simulink model "ackerman_ROS_controller_obstaculos_neuro_2022"  (R2022b)
settings: Solver=FixedStepDiscrete  StartTime=0.0  StopTime=120  FixedStep=0.1  RelTol=1e-3
undefined symbols (not defined in the file or in its folder): Angular, Linear
libraries: neural x78, robotlib x15, robotcorelib x1
(part 4 of 4)

== system ackerman_ROS_controller_obstaculos_neuro_2022/Feed-Forward Neural Network/Layer 3/Delays 1 ==
  "p{3}" : Inport  PortDimensions=20  SampleTime=0.1
      mask Display: e = 0.06;c1 = [120 230 180]/255;c2 = ([120 230 180]+0)/(256+128);c3 = ([120 230 180]+128)/(256+128);patch([0 1 1 0],[0 0 1 1],c1);patch([0 1 1 1-e 1-e 0+e],[0 0 1 1-e 0+e 0+e],c2);patch([0 0 1 1-e 0+e 0+e],[0 1 1 1-e 1-e 0+e],c3);plot([0 1 1 0 0],[0 0 1 1 0]);
  mux : Mux  Inputs=1
      mask Display: e = 0.06;c1 = [120 150 230]/255;c2 = ([120 150 230]+0)/383;c3 = ([120 150 230]+128)/383;patch([0 1 1 0],[0 0 1 1],c1);patch([0 1 1 1-e 1-e 0+e],[0 0 1 1-e 0+e 0+e],c2);patch([0 0 1 1-e 0+e 0+e],[0 1 1 1-e 1-e 0+e],c3);plot([0 1 1 0 0],[0 0 1 1 0]);disp('Mux')
  "pd{3,2}" : Outport
      mask Display: e = 0.06;c1 = [120 230 180]/255;c2 = ([120 230 180]+0)/(256+128);c3 = ([120 230 180]+128)/(256+128);patch([0 1 1 0],[0 0 1 1],c1);patch([0 1 1 1-e 1-e 0+e],[0 0 1 1-e 0+e 0+e],c2);patch([0 0 1 1-e 0+e 0+e],[0 1 1 1-e 1-e 0+e],c3);plot([0 1 1 0 0],[0 0 1 1 0]);
  wires:
  "p{3}"/1 -> mux/1
  mux/1 -> "pd{3,2}"/1

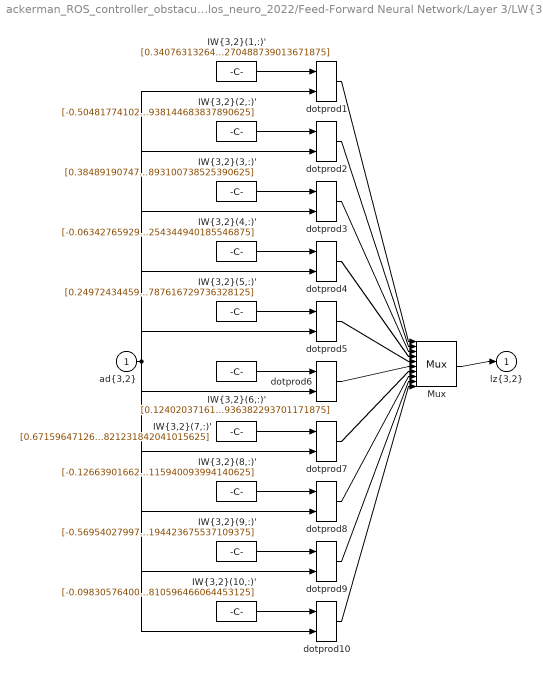
== system ackerman_ROS_controller_obstaculos_neuro_2022/Feed-Forward Neural Network/Layer 3/LW{3,2} ==
  "ad{3,2}" : Inport  PortDimensions=20  SampleTime=0.1
      mask Display: e = 0.06;c1 = [120 230 180]/255;c2 = ([120 230 180]+0)/(256+128);c3 = ([120 230 180]+128)/(256+128);patch([0 1 1 0],[0 0 1 1],c1);patch([0 1 1 1-e 1-e 0+e],[0 0 1 1-e 0+e 0+e],c2);patch([0 0 1 1-e 0+e 0+e],[0 1 1 1-e 1-e 0+e],c3);plot([0 1 1 0 0],[0 0 1 1 0]);
  "IW{3,2}(1,:)'" : Constant  Value=[0.34076313264394053614836366250528953969478607177734375;-0.7213416371848724306659050853340886533260345458984375;0.78614925426456261359220434314920566976070404052734375;-0.86204454200370861371993669308722019195556640625;-0.2285586359183717497511878491422976367175579071044921875;0.23760191269676855796433301293291151523590087890625;-0.251424166033277440845949968206696212291717529296875;-0.404852844355444274615507538328529335558414459228515625;0.13034380320936589381375370066962204873561859130859375;0.60706149796015618225197840729379095137119293212890625;0.57967174192335590987568139098584651947021484375;0.190902189478655170962184683958184905350208282470703125;-0.353602869044561174405316705815494060516357421875;0.5539034842942403003007711959071457386016845703125;0.35112311429221276792844719238928519189357757568359375;0.173037366849527141088316284367465414106845855712890625;0.28490880317578060054728439354221336543560028076171875;-0.28846529791194253089514631938072852790355682373046875;-0.6598111386363931796239512550528161227703094482421875;-0.1974712766146491105256899345476995222270488739013671875]
      mask Display: e = 0.06;c1 = [120 150 230]/255;c2 = ([120 150 230]+0)/383;c3 = ([120 150 230]+128)/383;patch([0 1 1 0],[0 0 1 1],c1);patch([0 1 1 1-e 1-e 0+e],[0 0 1 1-e 0+e 0+e],c2);patch([0 0 1 1-e 0+e 0+e],[0 1 1 1-e 1-e 0+e],c3);plot([0 1 1 0 0],[0 0 1 1 0]);disp('weights');
  "IW{3,2}(10,:)'" : Constant  Value=[-0.09830576400866973540981774704050621949136257171630859375;0.19584625654376264236589122447185218334197998046875;-0.07186883405932946444760744952873210422694683074951171875;-0.411132595147789547951333588571287691593170166015625;0.5587359300026497610502929092035628855228424072265625;-0.54956386482013208638619516932521946728229522705078125;0.96418797729135985452586510291439481079578399658203125;0.224205000801112053210317753837443888187408447265625;0.194211307244007425065746019754442386329174041748046875;0.1488208815166427445575436649960465729236602783203125;0.125350915148015162881023343288688920438289642333984375;-0.5560658230291941617196016522939316928386688232421875;0.63865397700167847450103408846189267933368682861328125;0.383742439241789912163227427299716509878635406494140625;-0.07663626948227875157471089551108889281749725341796875;0.308683270324817460306121574831195175647735595703125;0.0922442092653619483133553558218409307301044464111328125;0.28210419917956264246328146327869035303592681884765625;0.388901043212449171182498730559018440544605255126953125;0.4674781385723794091546778872725553810596466064453125]
      mask Display: e = 0.06;c1 = [120 150 230]/255;c2 = ([120 150 230]+0)/383;c3 = ([120 150 230]+128)/383;patch([0 1 1 0],[0 0 1 1],c1);patch([0 1 1 1-e 1-e 0+e],[0 0 1 1-e 0+e 0+e],c2);patch([0 0 1 1-e 0+e 0+e],[0 1 1 1-e 1-e 0+e],c3);plot([0 1 1 0 0],[0 0 1 1 0]);disp('weights');
  "IW{3,2}(2,:)'" : Constant  Value=[-0.504817741024414790018681742367334663867950439453125;-0.2228948316526042361385151480135391466319561004638671875;0.34074250793049165597636829261318780481815338134765625;-0.1272079004483044617490605787679669447243213653564453125;-0.421196726884725924922037165742949582636356353759765625;-0.423182365669241111749698802668717689812183380126953125;-0.64060323734867108402823987489682622253894805908203125;-0.41792590747442270870948277661227621138095855712890625;0.164025088337398872173622521586366929113864898681640625;0.000723803862171182831042326455417423858307301998138427734375;-0.37821645352981192456098824550281278789043426513671875;0.08450211339484814399014567243284545838832855224609375;0.54703156738828673244512401652173139154911041259765625;0.967854775030749348019298849976621568202972412109375;0.1959076268542807863770605081299436278641223907470703125;-0.87485126628045872809735783448559232056140899658203125;-0.56702287220650993138093554080114699900150299072265625;0.96608415914714462768841940487618558108806610107421875;0.28145560561015503520110314639168791472911834716796875;0.16213144910497911954649907784187234938144683837890625]
      mask Display: e = 0.06;c1 = [120 150 230]/255;c2 = ([120 150 230]+0)/383;c3 = ([120 150 230]+128)/383;patch([0 1 1 0],[0 0 1 1],c1);patch([0 1 1 1-e 1-e 0+e],[0 0 1 1-e 0+e 0+e],c2);patch([0 0 1 1-e 0+e 0+e],[0 1 1 1-e 1-e 0+e],c3);plot([0 1 1 0 0],[0 0 1 1 0]);disp('weights');
  "IW{3,2}(3,:)'" : Constant  Value=[0.38489190747757462407463435738463886082172393798828125;-0.269809596924946049067983722125063650310039520263671875;0.148592050165419820029200081989984028041362762451171875;0.13193229663022687514484232451650314033031463623046875;0.6417085342484594168155354054761119186878204345703125;-0.085986814940040512400543093463056720793247222900390625;0.55278354356485992493475123410462401807308197021484375;-0.00514271427792319969773959797976203844882547855377197265625;0.214148262828940449953307734176632948219776153564453125;0.49129027017042192770901465337374247610569000244140625;-0.867172068222769265588567577651701867580413818359375;-0.2580297917727190082359811640344560146331787109375;-0.296787967449555434296115663528325967490673065185546875;0.1761779750019051016263205156064941547811031341552734375;-0.0442969572291785074202863370373961515724658966064453125;0.334057171474406777722521155737922526895999908447265625;0.50279858245511632741653329503606073558330535888671875;-0.42466518553253485013243562207208015024662017822265625;0.312245093426585962337327373461448587477207183837890625;-0.679193415415080270491898772888816893100738525390625]
      mask Display: e = 0.06;c1 = [120 150 230]/255;c2 = ([120 150 230]+0)/383;c3 = ([120 150 230]+128)/383;patch([0 1 1 0],[0 0 1 1],c1);patch([0 1 1 1-e 1-e 0+e],[0 0 1 1-e 0+e 0+e],c2);patch([0 0 1 1-e 0+e 0+e],[0 1 1 1-e 1-e 0+e],c3);plot([0 1 1 0 0],[0 0 1 1 0]);disp('weights');
  "IW{3,2}(4,:)'" : Constant  Value=[-0.06342765929404418911996543783970992080867290496826171875;-0.453108556467711143245225002829101867973804473876953125;-0.054283585200033568352040447280160151422023773193359375;0.49124703787862900039584701517014764249324798583984375;-0.7060637807386758169059248757548630237579345703125;-0.00324291179714940314138260646359412930905818939208984375;1.1175411962726971015769095174618996679782867431640625;-0.162682966034998710558312495777499862015247344970703125;-0.42628897980284985447241297151776961982250213623046875;0.07672565387939282721685430033176089636981487274169921875;0.7384068836400425883681464256369508802890777587890625;0.376231060623061719372373090664041228592395782470703125;0.51842445167443773623716651854920201003551483154296875;-0.4914225121977102705983497799024917185306549072265625;0.10865284681541030609164266707011847756803035736083984375;-0.2438826420138709150098321742916596122086048126220703125;-0.101528735981841033986228239882620982825756072998046875;0.1146187243870478156271275338440318591892719268798828125;-0.797131570303906134000726524391211569309234619140625;-0.64041166823470785374183833482675254344940185546875]
      mask Display: e = 0.06;c1 = [120 150 230]/255;c2 = ([120 150 230]+0)/383;c3 = ([120 150 230]+128)/383;patch([0 1 1 0],[0 0 1 1],c1);patch([0 1 1 1-e 1-e 0+e],[0 0 1 1-e 0+e 0+e],c2);patch([0 0 1 1-e 0+e 0+e],[0 1 1 1-e 1-e 0+e],c3);plot([0 1 1 0 0],[0 0 1 1 0]);disp('weights');
  "IW{3,2}(5,:)'" : Constant  Value=[0.2497243445919992421710986718608182854950428009033203125;0.56882233095299827851931695477105677127838134765625;-0.445927445428407731586872841944568790495395660400390625;-0.360454610574551137514021093011251650750637054443359375;0.2283933175789964187263336725663975812494754791259765625;-0.275409819990113768906070390585227869451045989990234375;-0.58421622808207074317721207989961840212345123291015625;0.192441164478787396507897256014985032379627227783203125;-0.46791742141683434486054693479673005640506744384765625;1.0537604641889259937670431099832057952880859375;0.178736145372547505782989674116834066808223724365234375;-0.50159954482332824721169117765384726226329803466796875;0.6129068653836728941541878157295286655426025390625;0.539618571470044994242698521702550351619720458984375;0.513017753087568362246884134947322309017181396484375;0.231639287328622600625749328173696994781494140625;-0.33410826953662209337636568307061679661273956298828125;0.483221828394903629710910308858728967607021331787109375;-0.28077252670323316063871743608615361154079437255859375;0.00394198138773049766570011342992074787616729736328125]
      mask Display: e = 0.06;c1 = [120 150 230]/255;c2 = ([120 150 230]+0)/383;c3 = ([120 150 230]+128)/383;patch([0 1 1 0],[0 0 1 1],c1);patch([0 1 1 1-e 1-e 0+e],[0 0 1 1-e 0+e 0+e],c2);patch([0 0 1 1-e 0+e 0+e],[0 1 1 1-e 1-e 0+e],c3);plot([0 1 1 0 0],[0 0 1 1 0]);disp('weights');
  "IW{3,2}(6,:)'" : Constant  Value=[0.12402037161954858335288776061133830808103084564208984375;0.54132558115768525386357623574440367519855499267578125;-0.150636817909798548242861215840093791484832763671875;0.2048985139329151106135640247885021381080150604248046875;-0.470383253604719886453722210717387497425079345703125;-0.181244073381964465596638547140173614025115966796875;0.97978681625116836872990688789286650717258453369140625;-0.31941252858621937971150828161626122891902923583984375;-0.402473151915626659036462342555751092731952667236328125;-0.075314336408769333441881599355838261544704437255859375;0.25383510033730105615035199662088416516780853271484375;-0.10162216139321299246400798210743232630193233489990234375;0.124208043035973825229945077808224596083164215087890625;0.95664486089769862342535589050385169684886932373046875;-0.18687860383802490371607518682139925658702850341796875;0.09135665326397350571863142931761103682219982147216796875;0.7691219480882820480616146596730686724185943603515625;0.461061268580249483672872656825347803533077239990234375;0.235872592435734329541219267412088811397552490234375;-1.2150510338650846176022923827986232936382293701171875]
      mask Display: e = 0.06;c1 = [120 150 230]/255;c2 = ([120 150 230]+0)/383;c3 = ([120 150 230]+128)/383;patch([0 1 1 0],[0 0 1 1],c1);patch([0 1 1 1-e 1-e 0+e],[0 0 1 1-e 0+e 0+e],c2);patch([0 0 1 1-e 0+e 0+e],[0 1 1 1-e 1-e 0+e],c3);plot([0 1 1 0 0],[0 0 1 1 0]);disp('weights');
  "IW{3,2}(7,:)'" : Constant  Value=[0.67159647126277766115975964567041955888271331787109375;0.00430220644823856197824785141392567311413586139678955078125;0.370374570807203540301344446561415679752826690673828125;0.5053222240793282526993834835593588650226593017578125;0.42776647463469907872735120690776966512203216552734375;0.278472194666314842859122791196568869054317474365234375;0.29359921607298000711949725882732309401035308837890625;-0.3184392319202780097242566625936888158321380615234375;0.06723219890412902854937016172698349691927433013916015625;0.397552363692675270190335368170053698122501373291015625;-0.73981614880413371082568119163624942302703857421875;-0.34122180921187894586665834140148945152759552001953125;-0.490456665996303164956060527401859872043132781982421875;-0.1386466910442335220832177355987369082868099212646484375;0.2146983586610520522430789469581213779747486114501953125;-0.0041578847732147393434498638953300542198121547698974609375;-0.3806092490588259824590977586922235786914825439453125;0.0953799197057930425724947554044774733483791351318359375;0.496643356283201387046943864334025420248508453369140625;-0.119304835550778476349620405017049051821231842041015625]
      mask Display: e = 0.06;c1 = [120 150 230]/255;c2 = ([120 150 230]+0)/383;c3 = ([120 150 230]+128)/383;patch([0 1 1 0],[0 0 1 1],c1);patch([0 1 1 1-e 1-e 0+e],[0 0 1 1-e 0+e 0+e],c2);patch([0 0 1 1-e 0+e 0+e],[0 1 1 1-e 1-e 0+e],c3);plot([0 1 1 0 0],[0 0 1 1 0]);disp('weights');
  "IW{3,2}(8,:)'" : Constant  Value=[-0.1266390166226174784913638404759694822132587432861328125;0.1346511877306488524919103610955062322318553924560546875;0.1704886432583949951169444148035836406052112579345703125;-1.663131542922095196246345949475653469562530517578125;-0.257204106916682884165226141703897155821323394775390625;0.126240724847572372002701968085602857172489166259765625;0.462680862814355997603144032837008126080036163330078125;-0.0731964798157098972541945158809539861977100372314453125;0.1061116292981826580987814168111071921885013580322265625;0.1795995958768095424051836062062648124992847442626953125;-0.1988701276775927950790645581946591846644878387451171875;0.06830386534616005034248331639901152811944484710693359375;0.5265929386354437635731073896749876439571380615234375;0.245497291327573086139324232135550118982791900634765625;1.19165268537236013202118556364439427852630615234375;-0.1477242295209958145019157882416038773953914642333984375;-1.4425074165352038679799306919449009001255035400390625;0.00022506382979615990880262188511551357805728912353515625;-0.2281389132459103741279449195644701831042766571044921875;0.1088713090552137219280126601006486453115940093994140625]
      mask Display: e = 0.06;c1 = [120 150 230]/255;c2 = ([120 150 230]+0)/383;c3 = ([120 150 230]+128)/383;patch([0 1 1 0],[0 0 1 1],c1);patch([0 1 1 1-e 1-e 0+e],[0 0 1 1-e 0+e 0+e],c2);patch([0 0 1 1-e 0+e 0+e],[0 1 1 1-e 1-e 0+e],c3);plot([0 1 1 0 0],[0 0 1 1 0]);disp('weights');
  "IW{3,2}(9,:)'" : Constant  Value=[-0.569540279977478913764343815273605287075042724609375;0.36417437716836598138314684547367505729198455810546875;-0.5343836970062285640636901007383130490779876708984375;-0.39444339607602085795434732062858529388904571533203125;-0.0134222854716614277414965528123502735979855060577392578125;0.57867912879174088214284665809827856719493865966796875;-0.06092514543647147007288111808520625345408916473388671875;-0.046768935366277165910364743695026845671236515045166015625;-0.469529752777478937009192350160446949303150177001953125;-0.1304864270836427753152975128614343702793121337890625;-0.0745117698762659264044572182683623395860195159912109375;0.49898106776690565045129233112675137817859649658203125;-0.162143371121196311346324137048213742673397064208984375;0.25585127581901734306057960566249676048755645751953125;0.671614452905421099870864054537378251552581787109375;-0.230931487991691442029917880063294433057308197021484375;-0.4173399864363516176268831259221769869327545166015625;0.177450052743841180102890575653873383998870849609375;0.002833560094522368823233282597584548057056963443756103515625;0.109620670516186569098948666578507982194423675537109375]
      mask Display: e = 0.06;c1 = [120 150 230]/255;c2 = ([120 150 230]+0)/383;c3 = ([120 150 230]+128)/383;patch([0 1 1 0],[0 0 1 1],c1);patch([0 1 1 1-e 1-e 0+e],[0 0 1 1-e 0+e 0+e],c2);patch([0 0 1 1-e 0+e 0+e],[0 1 1 1-e 1-e 0+e],c3);plot([0 1 1 0 0],[0 0 1 1 0]);disp('weights');
  Mux : Mux  Inputs=10
      mask Display: e = 0.06;c1 = [120 150 230]/255;c2 = ([120 150 230]+0)/383;c3 = ([120 150 230]+128)/383;patch([0 1 1 0],[0 0 1 1],c1);patch([0 1 1 1-e 1-e 0+e],[0 0 1 1-e 0+e 0+e],c2);patch([0 0 1 1-e 0+e 0+e],[0 1 1 1-e 1-e 0+e],c3);plot([0 1 1 0 0],[0 0 1 1 0]);disp('Mux');
  dotprod{1..10} (10 alike) : neural/Weight Functions/dotprod
  "lz{3,2}" : Outport
      mask Display: e = 0.06;c1 = [120 230 180]/255;c2 = ([120 230 180]+0)/(256+128);c3 = ([120 230 180]+128)/(256+128);patch([0 1 1 0],[0 0 1 1],c1);patch([0 1 1 1-e 1-e 0+e],[0 0 1 1-e 0+e 0+e],c2);patch([0 0 1 1-e 0+e 0+e],[0 1 1 1-e 1-e 0+e],c3);plot([0 1 1 0 0],[0 0 1 1 0]);
  wires:
  "IW{3,2}(1,:)'"/1 -> dotprod1/1
  "ad{3,2}"/1 -> dotprod1/2, dotprod2/2, dotprod3/2, dotprod4/2, dotprod5/2, dotprod6/2, dotprod7/2, dotprod8/2, dotprod9/2, dotprod10/2
  dotprod1/1 -> Mux/1
  "IW{3,2}(2,:)'"/1 -> dotprod2/1
  dotprod2/1 -> Mux/2
  "IW{3,2}(3,:)'"/1 -> dotprod3/1
  dotprod3/1 -> Mux/3
  "IW{3,2}(4,:)'"/1 -> dotprod4/1
  dotprod4/1 -> Mux/4
  "IW{3,2}(5,:)'"/1 -> dotprod5/1
  dotprod5/1 -> Mux/5
  "IW{3,2}(6,:)'"/1 -> dotprod6/1
  dotprod6/1 -> Mux/6
  "IW{3,2}(7,:)'"/1 -> dotprod7/1
  dotprod7/1 -> Mux/7
  "IW{3,2}(8,:)'"/1 -> dotprod8/1
  dotprod8/1 -> Mux/8
  "IW{3,2}(9,:)'"/1 -> dotprod9/1
  dotprod9/1 -> Mux/9
  "IW{3,2}(10,:)'"/1 -> dotprod10/1
  dotprod10/1 -> Mux/10
  Mux/1 -> "lz{3,2}"/1

== system ackerman_ROS_controller_obstaculos_neuro_2022/Feed-Forward Neural Network/Layer 4/Delays 1 ==
  "p{4}" : Inport  PortDimensions=10  SampleTime=0.1
      mask Display: e = 0.06;c1 = [120 230 180]/255;c2 = ([120 230 180]+0)/(256+128);c3 = ([120 230 180]+128)/(256+128);patch([0 1 1 0],[0 0 1 1],c1);patch([0 1 1 1-e 1-e 0+e],[0 0 1 1-e 0+e 0+e],c2);patch([0 0 1 1-e 0+e 0+e],[0 1 1 1-e 1-e 0+e],c3);plot([0 1 1 0 0],[0 0 1 1 0]);
  mux : Mux  Inputs=1
      mask Display: e = 0.06;c1 = [120 150 230]/255;c2 = ([120 150 230]+0)/383;c3 = ([120 150 230]+128)/383;patch([0 1 1 0],[0 0 1 1],c1);patch([0 1 1 1-e 1-e 0+e],[0 0 1 1-e 0+e 0+e],c2);patch([0 0 1 1-e 0+e 0+e],[0 1 1 1-e 1-e 0+e],c3);plot([0 1 1 0 0],[0 0 1 1 0]);disp('Mux')
  "pd{4,3}" : Outport
      mask Display: e = 0.06;c1 = [120 230 180]/255;c2 = ([120 230 180]+0)/(256+128);c3 = ([120 230 180]+128)/(256+128);patch([0 1 1 0],[0 0 1 1],c1);patch([0 1 1 1-e 1-e 0+e],[0 0 1 1-e 0+e 0+e],c2);patch([0 0 1 1-e 0+e 0+e],[0 1 1 1-e 1-e 0+e],c3);plot([0 1 1 0 0],[0 0 1 1 0]);
  wires:
  "p{4}"/1 -> mux/1
  mux/1 -> "pd{4,3}"/1

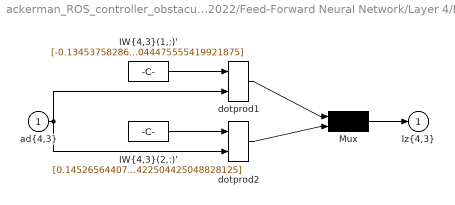
== system ackerman_ROS_controller_obstaculos_neuro_2022/Feed-Forward Neural Network/Layer 4/LW{4,3} ==
  "ad{4,3}" : Inport  PortDimensions=10  SampleTime=0.1
      mask Display: e = 0.06;c1 = [120 230 180]/255;c2 = ([120 230 180]+0)/(256+128);c3 = ([120 230 180]+128)/(256+128);patch([0 1 1 0],[0 0 1 1],c1);patch([0 1 1 1-e 1-e 0+e],[0 0 1 1-e 0+e 0+e],c2);patch([0 0 1 1-e 0+e 0+e],[0 1 1 1-e 1-e 0+e],c3);plot([0 1 1 0 0],[0 0 1 1 0]);
  "IW{4,3}(1,:)'" : Constant  Value=[-0.1345375828613024349333926465988042764365673065185546875;0.1233915526277311880409826017057639546692371368408203125;-0.12186700394563033944539398589768097735941410064697265625;0.352917537927395608132741244844510219991207122802734375;-0.0993644045013619414685734909653547219932079315185546875;-0.135764938772570786795768071897327899932861328125;-0.288083370306218722323166048226994462311267852783203125;-0.61929246006747196151565049149212427437305450439453125;-0.29376035043953752090573061650502495467662811279296875;-0.34392461894868098237765252633835189044475555419921875]
      mask Display: e = 0.06;c1 = [120 150 230]/255;c2 = ([120 150 230]+0)/383;c3 = ([120 150 230]+128)/383;patch([0 1 1 0],[0 0 1 1],c1);patch([0 1 1 1-e 1-e 0+e],[0 0 1 1-e 0+e 0+e],c2);patch([0 0 1 1-e 0+e 0+e],[0 1 1 1-e 1-e 0+e],c3);plot([0 1 1 0 0],[0 0 1 1 0]);disp('weights');
  "IW{4,3}(2,:)'" : Constant  Value=[0.1452656440752886635170426643526297993957996368408203125;-0.0729163710939332021521153137655346654355525970458984375;0.2476384278400275695819487964399741031229496002197265625;-0.2472976244973816850603043349110521376132965087890625;-0.509905304132805436978514990187250077724456787109375;-0.147706754520010641318350508299772627651691436767578125;0.1894797338716689427684514157590456306934356689453125;0.338980287317378559119873671079403720796108245849609375;0.95598991402642552461799141383380629122257232666015625;0.353070088191287212442404097600956447422504425048828125]
      mask Display: e = 0.06;c1 = [120 150 230]/255;c2 = ([120 150 230]+0)/383;c3 = ([120 150 230]+128)/383;patch([0 1 1 0],[0 0 1 1],c1);patch([0 1 1 1-e 1-e 0+e],[0 0 1 1-e 0+e 0+e],c2);patch([0 0 1 1-e 0+e 0+e],[0 1 1 1-e 1-e 0+e],c3);plot([0 1 1 0 0],[0 0 1 1 0]);disp('weights');
  Mux : Mux  Inputs=2
      mask Display: e = 0.06;c1 = [120 150 230]/255;c2 = ([120 150 230]+0)/383;c3 = ([120 150 230]+128)/383;patch([0 1 1 0],[0 0 1 1],c1);patch([0 1 1 1-e 1-e 0+e],[0 0 1 1-e 0+e 0+e],c2);patch([0 0 1 1-e 0+e 0+e],[0 1 1 1-e 1-e 0+e],c3);plot([0 1 1 0 0],[0 0 1 1 0]);disp('Mux');
  dotprod1 : neural/Weight Functions/dotprod
  dotprod2 : neural/Weight Functions/dotprod
  "lz{4,3}" : Outport
      mask Display: e = 0.06;c1 = [120 230 180]/255;c2 = ([120 230 180]+0)/(256+128);c3 = ([120 230 180]+128)/(256+128);patch([0 1 1 0],[0 0 1 1],c1);patch([0 1 1 1-e 1-e 0+e],[0 0 1 1-e 0+e 0+e],c2);patch([0 0 1 1-e 0+e 0+e],[0 1 1 1-e 1-e 0+e],c3);plot([0 1 1 0 0],[0 0 1 1 0]);
  wires:
  "IW{4,3}(1,:)'"/1 -> dotprod1/1
  "ad{4,3}"/1 -> dotprod1/2, dotprod2/2
  dotprod1/1 -> Mux/1
  "IW{4,3}(2,:)'"/1 -> dotprod2/1
  dotprod2/1 -> Mux/2
  Mux/1 -> "lz{4,3}"/1

== matlab function ackerman_ROS_controller_obstaculos_neuro_2022/ROS Robot/Conversion_diff_ackerman ==
  data: steering_wheel_angle input; V output; linear_vel_ackerman_kmh input; W output
function [V,W] = fcn(steering_wheel_angle, linear_vel_ackerman_kmh)

    %Aproximacion de angulo volante y velocidad linal a vel_linar y angular.
    % *************************************
    
    min_turning_radius_vehicle = 2;  % radio de giro del vehiculo. Radio minimo en el que gira 180 grados. 
    max_turning_radius_vehicle = 34; % radio de giro del vehiculo. Radio máximo con el volante girado 1º
    max_steering_wheel_angle = 90;  % angulo máximo de volante permitido (grados).
    max_vehicle_linear_speed = 50;  % velocidad máxima de vehiculo (km/h).
    
    
    % Filtrado des los valores máximos
    
    if steering_wheel_angle > max_steering_wheel_angle
        steering_wheel_angle = max_steering_wheel_angle;  
    end
    
    if steering_wheel_angle < (-1*max_steering_wheel_angle)
        steering_wheel_angle = max_steering_wheel_angle;  
    end
    
    if linear_vel_ackerman_kmh > max_vehicle_linear_speed
        linear_vel_ackerman_kmh = max_vehicle_linear_speed;
    end
    
    
    %Conversion a m/s
    linear_vel_ackerman_ms = linear_vel_ackerman_kmh/3.6; %(m/s)
    
    %Conversion a linear and angular velocity for the simulator.
    % v=rω --> ω = v/r
    
    % max_steering_wheel_angle -- > min_turning_radius_vehicle
    % steering_wheel_angle = 0 --> angular_vel_vehicle = 0;
    
    turning_radius = (max_turning_radius_vehicle-((max_turning_radius_vehicle-min_turning_radius_vehicle)/max_steering_wheel_angle)*abs(steering_wheel_angle));
    
    if steering_wheel_angle > 0
            turning_radius = turning_radius;
    elseif steering_wheel_angle < 0
            turning_radius = -1*turning_radius;
    end
    
    if abs(steering_wheel_angle) < 0.01
        angular_vel_vehicle = 0;
    else
        angular_vel_vehicle = linear_vel_ackerman_ms / turning_radius;
    end
    
    %Sin velocidad linear, tampoco debe girar
    
    if linear_vel_ackerman_ms == 0
        angular_vel_vehicle = 0;
    end
    
    
    %Rellenamos los campos del mensaje V y W
    V= linear_vel_ackerman_ms;

    W=angular_vel_vehicle;
    
    
    %********************************************************

== matlab function ackerman_ROS_controller_obstaculos_neuro_2022/ROS Robot/MATLAB Function ==
  data: u input; y output
function y = fcn(u)
u(isinf(u))=15.0;
y = u;

== matlab function ackerman_ROS_controller_obstaculos_neuro_2022/MATLAB Function ==
  data: stop_flag input; vel output; vel input; steering_wheel input; steering_wheel output
function [vel, steering_wheel]= stop(stop_flag,vel,steering_wheel)
    if stop_flag 
        steering_wheel=0;
        vel=0;
    else
        vel=vel;
        steering_wheel=steering_wheel;
    end

== matlab function ackerman_ROS_controller_obstaculos_neuro_2022/Evaluacion_maniobra/evaluacion_fin ==
  data: clock input; x input; y input; theta input; stop_flag output
function stop_flag = evaluacion_fin(clock, x, y, theta)
    if x > 59 && x < 60
        if y < 4
            stop_flag = 1;
        else 
            stop_flag = 0;
        end
        else
            stop_flag = 0;
    end
end
